simulink model "sf_combined_state_actions"  (Simulink 7.6)
settings: Solver=FixedStepDiscrete  StartTime=0.0  StopTime=5.0  RelTol=1e-3
settings Model: Creator=The MathWorks Inc.
settings DebuggingCC: SolverPrmCheckMsg=none
settings SFSimCC: SimParseCustomCode=off

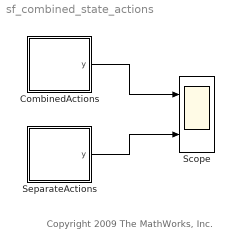
== system sf_combined_state_actions ==
  note: Copyright 2009 The MathWorks, Inc.
  CombinedActions : Stateflow chart  TreatAsAtomicUnit=on
  Scope : Scope  NumInputPorts=2
      settings: TimeRange=5  YMin=0~0  YMax=8~8
  SeparateActions : Stateflow chart  TreatAsAtomicUnit=on
  wires:
  CombinedActions/1(y) -> Scope/1
  SeparateActions/1(y) -> Scope/2

== stateflow chart CombinedActions ==
  state A
    en: y=0;
    en, du: y++;
  state B
  (default) -> A
  A -> B : after(5,tick)
  data: y output double

== stateflow chart SeparateActions ==
  state A
    en: y=0;
    en: y++;
    du: y++;
  state B
  (default) -> A
  A -> B : after(5,tick)
  data: y output double
